simulink model "Battery_test"  (R2016b)
settings: Solver=FixedStepAuto  StartTime=0.0  StopTime=3600  FixedStep=10  RelTol=1e-3
values from neighbouring files (symbols this model uses):
  bat_energy = bat_energy_kwh*1000*3600    (= 216000000)    [Init_PI_reg.m]    (also in Initial_test.m; battery_test_res.mat; body_test_res.mat; motor_test_res.mat)
  R_dc = 0.25    [Init_PI_reg.m]    (also in Initial_test.m; battery_test_res.mat; body_test_res.mat; motor_test_res.mat)
  soc = [0, 2, 6, 9, 20, 37, 42, 57, 66, 77, 85, 91, 95, 98, 100]    [Init_PI_reg.m]    (also in Initial_test.m; battery_test_res.mat = [0 2 6 9 20 37 42 57 66 77 85 91 ... (15 elements, 1x15)]; body_test_res.mat = [0 2 6 9 20 37 42 57 66 77 85 91 ... (15 elements, 1x15)]; motor_test_res.mat = [0 2 6 9 20 37 42 57 66 77 85 91 ... (15 elements, 1x15)])
  U_bat = U_cell*Nb_serial    [Init_PI_reg.m]    (also in Initial_test.m; battery_test_res.mat = [327.36 346.56 362.88 370.56 373.44 374.4 376.32 381.12 384 ; body_test_res.mat = [327.36 346.56 362.88 370.56 373.44 374.4 376.32 381.12 384 ; motor_test_res.mat = [327.36 346.56 362.88 370.56 373.44 374.4 376.32 381.12 384 )
libraries: simulink x1
settings Model: Creator=a037702  LastModifiedBy=a037702

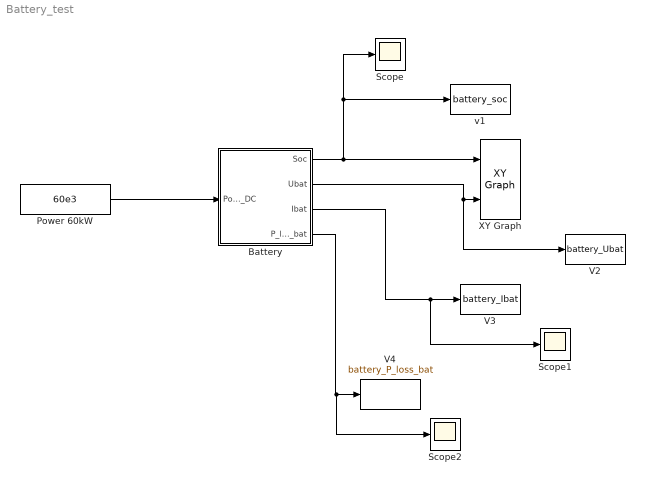
== system Battery_test ==
  Battery : Subsystem
  Power 60kW : Constant  Value=60e3
  Scope : Scope
  Scope1 : Scope
  Scope2 : Scope
  V2 : ToWorkspace  VariableName=battery_Ubat  SaveFormat=Structure With Time  SampleTime=-1
      settings: Save2DSignal=2-D array (concatenate along first dimension)
  V3 : ToWorkspace  VariableName=battery_Ibat  SaveFormat=Structure With Time  SampleTime=-1
      settings: Save2DSignal=2-D array (concatenate along first dimension)
  V4 : ToWorkspace  VariableName=battery_P_loss_bat  SaveFormat=Structure With Time  SampleTime=-1
      settings: Save2DSignal=2-D array (concatenate along first dimension)
  XY Graph : simulink/Sinks/XY Graph  xmin=-inf  xmax=inf  ymin=-inf  ymax=inf  st=-1
  v1 : ToWorkspace  VariableName=battery_soc  SaveFormat=Structure With Time  SampleTime=-1
      settings: Save2DSignal=2-D array (concatenate along first dimension)
  wires:
  Battery/1(Soc) -> XY Graph/1, v1/1, Scope/1
  Battery/2(Ubat) -> V2/1, XY Graph/2
  Power 60kW/1 -> Battery/1(Power_DC)
  Battery/3(Ibat) -> Scope1/1, V3/1
  Battery/4(P_loss_bat) -> Scope2/1, V4/1

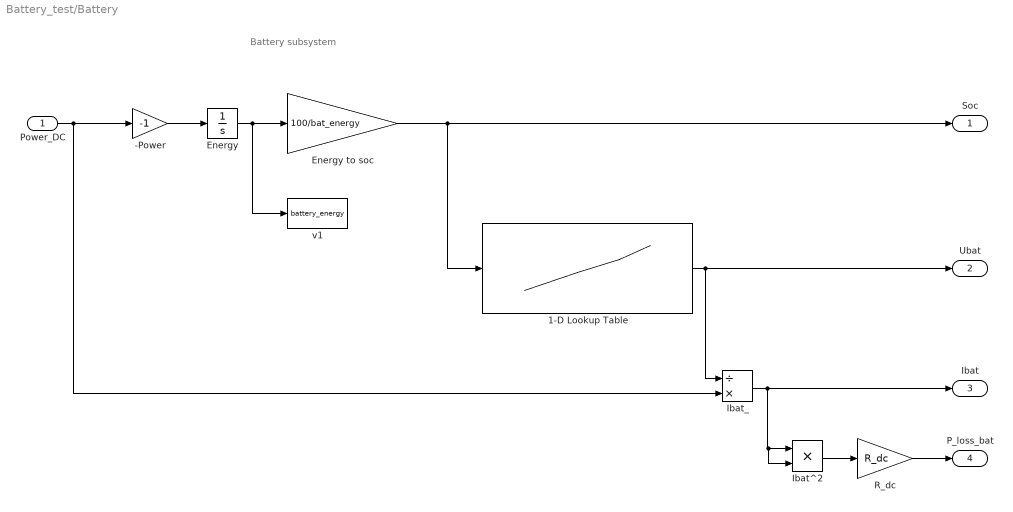
== system Battery_test/Battery ==
  note: Battery subsystem
  Power_DC : Inport
  -Power : Gain  Gain=-1
  1-D Lookup Table : Lookup_n-D  NumberOfTableDimensions=1  BreakpointsForDimension1=soc  BreakpointsForDimension1DataTypeStr=double  Table=U_bat  TableDataTypeStr=double  InternalRulePriority=Speed  RndMeth=Simplest  InputSameDT=on
  Energy : Integrator  InitialCondition=bat_energy  LimitOutput=on  UpperSaturationLimit=bat_energy  LowerSaturationLimit=0
  Energy to soc : Gain  Gain=100/bat_energy
  Ibat^2 : Product  Inputs=**
  Ibat_ : Product  Inputs=/*
  R_dc : Gain  Gain=R_dc
  v1 : ToWorkspace  VariableName=battery_energy  SaveFormat=Structure With Time  SampleTime=-1
      settings: Save2DSignal=2-D array (concatenate along first dimension)
  Soc : Outport
  Ubat : Outport  Port=2
  Ibat : Outport  Port=3
  P_loss_bat : Outport  Port=4
  wires:
  Energy/1 -> v1/1, Energy to soc/1
  Energy to soc/1 -> 1-D Lookup Table/1, Soc/1
  Power_DC/1 -> Ibat_/2, -Power/1
  1-D Lookup Table/1 -> Ibat_/1, Ubat/1
  Ibat_/1 -> Ibat^2/2, Ibat^2/1, Ibat/1
  Ibat^2/1 -> R_dc/1
  R_dc/1 -> P_loss_bat/1
  -Power/1 -> Energy/1
